simulink model "model_5LinkWalking"  (R2022b)
settings: Solver=ode45  StartTime=0.0  StopTime=Tf  FixedStep=1e-5  MaxStep=1e-3  RelTol=1e-12  AbsTol=1e-8
values from neighbouring files (symbols this model uses):
  f_dist = [0; -100; 0]    [main.m]    (also in main_5linkWalking_PSO.m)
  gains = [ ... (first row only)    [main.m]    (also in main_5linkWalking_PSO.m = [gain.kP1, gain.kD1, gain.kP2, gain.kD2, gain.kP3, gain.kD3,)
  gains_VSLIPSL = [gain_VSLIPSL.K_p; gain_VSLIPSL.K_d; gain_VSLIPSL.K_p_sw; gain_VSLIPSL.K_d_sw; gain_VSLIPSL.K_p_ds; gain_VSLIPSL.K_d_ds; gain_VSLIPSL.K_v_ds]    [main.m]    (also in main_5linkWalking_PSO.m)
  init_flag = [1; 0; -dc.col_param.footPlus; -slipsl.time_ss(N); slipsl.x_ss(1); slipsl.y_ss(1); alpha_ss_ref(1)]    [main.m]    (also in main_5linkWalking_PSO.m = [1; 0; -dc.col_param.footPlus; 0; CoM(1); CoM(2)])
  Initial_state = [q0;dq0]    [main.m]    (also in main_5linkWalking_PSO.m)
  param = [params.m1; params.m2; params.m5; params.l1; params.l2; params.l5; params.g; params.I1; params.I2; params.I5; params.r_k; params.r_h; params.k_ba; params.phi_h0; params.phi_k0]    [main.m]    (also in main_5linkWalking_PSO.m = [params.m1; params.m2; params.m5; params.l1; params.l2; para)
  ref_star_ds = [ref_star.ds.x_CoM_star,      ref_star.ds.y_CoM_star, ref_star.ds.dx_CoM_star,      ref_star.ds.del_y_CoM_star, ref_star.ds.del_dx_CoM_star,      ref_star.ds.del2_y_CoM_star]    [main.m]    (also in main_5linkWalking_PSO.m)
  ref_star_ss = [ref_star.ss.x_M_star,      ref_star.ss.y_M_star, ref_star.ss.x_swFoot_star, ref_star.ss.y_swFoot_star,      ref_star.ss.del_y_M_star, ref_star.ss.del_x_swFoot_star, ref_star.ss.del_y_swFoot_star,      ref_star.ss.del2_y_M_star, ref_star.ss.del2_x_swFoot_star, ref_star.ss.del2_y_swFoot_star,      ref_star.ss.x_CoM_star]    [main.m]    (also in main_5linkWalking_PSO.m)
  sample_time = 0.001    [main.m]    (also in main_5linkWalking_PSO.m)
  slipslParams = [ ... (first row only)    [main.m]    (also in main_5linkWalking_PSO.m)
  slipslTraj_ds = [slipsl.time_ds, slipsl.x_ds, slipsl.y_ds, slipsl.dx_ds, slipsl.dy_ds, alpha_ds_ref_discrete]    [main.m]    (also in main_5linkWalking_PSO.m = [ref_star.dc.ds.time - ref_star.dc.ds.time(1), ref_star.dc.d)
  slipslTraj_ss = [slipsl.time_ss, slipsl.x_ss, slipsl.y_ss, slipsl.dx_ss, slipsl.dy_ss, alpha_ss_ref_discrete]    [main.m]    (also in main_5linkWalking_PSO.m = [ref_star.dc.ss.time, ref_star.dc.ss.x_CoM', ref_star.dc.ss.)
  swFootTraj = [swFootSLIPSL.x_CoM, swFootSLIPSL.x, swFootSLIPSL.z, swFootSLIPSL.dx, swFootSLIPSL.dz]    [main.m]    (also in main_5linkWalking_PSO.m = [ref_star.dc.ss.x_CoM', ref_star.dc.ss.x_sw', ref_star.dc.ss)
libraries: simulink x1
(part 3 of 3)

== matlab function model_5LinkWalking/Model dynamics/STOP system when dx_CoM<=0/MATLAB Function ==
  data: u input
function fcn(u)
if u ~= 0
    disp('dx < 0')
end

== matlab function model_5LinkWalking/Model dynamics/Continuous dynamics ==
  data: t input; U input; dX output; rec_cs_force output; X input; param input; flg_VLO output; flag input; CoM_acc output; f_dist input
function [dX, rec_cs_force, flg_VLO, CoM_acc] = fcn(t, U, X, param, flag, f_dist)

%% variables
th1 = X(1);
th2 = X(2);
th3 = X(3);
th4 = X(4);
th5 = X(5);

dth1 = X(6);
dth2 = X(7);
dth3 = X(8);
dth4 = X(9);
dth5 = X(10);

q = [th1;th2;th3;th4;th5];
dq = [dth1;dth2;dth3;dth4;dth5];

%% parameters

m1 = param(1);
m2 = param(2);
m3 = m2;
m4 = m1;
m5 = param(3);

l1 = param(4);
l2 = param(5);
l5 = param(6);
l3 = l2;
l4 = l1;

gravi = param(7);
I1 = param(8);
I2 = param(9);
I5 = param(10);
I3 = I1;
I4 = I2;

%% flags
f_SS = flag(1); % indicates which stance phase it is
foot = flag(2); % location of the stance foot
foot_prev = flag(3); % previous location of the stance foot

%% Inertia Matrix
MM = MM_matrix(X,param);

%% Centrifugal force · Coriolis force Vector
CC = zeros(5,1);

CC(1, 1) = - (dth2^2*l1*l3*m3*sin(th2 + th3))/2 - dth2^2*l1*l3*m4*sin(th2 + th3) - (dth3^2*l1*l3*m3*sin(th2 + th3))/2 - dth3^2*l1*l3*m4*sin(th2 + th3) - (dth2^2*l1*l5*m5*sin(th2 + th5))/2 - (dth3^2*l2*l4*m4*sin(th3 + th4))/2 - (dth4^2*l2*l4*m4*sin(th3 + th4))/2 - (dth5^2*l1*l5*m5*sin(th2 + th5))/2 - (dth2^2*l1*l2*m2*sin(th2))/2 - dth2^2*l1*l2*m3*sin(th2) - dth2^2*l1*l2*m4*sin(th2) - dth2^2*l1*l2*m5*sin(th2) - (dth3^2*l2*l3*m3*sin(th3))/2 - dth3^2*l2*l3*m4*sin(th3) - (dth4^2*l3*l4*m4*sin(th4))/2 - (dth5^2*l2*l5*m5*sin(th5))/2 - (dth2^2*l1*l4*m4*sin(th2 + th3 + th4))/2 - (dth3^2*l1*l4*m4*sin(th2 + th3 + th4))/2 - (dth4^2*l1*l4*m4*sin(th2 + th3 + th4))/2 - dth1*dth2*l1*l3*m3*sin(th2 + th3) - 2*dth1*dth2*l1*l3*m4*sin(th2 + th3) - dth1*dth3*l1*l3*m3*sin(th2 + th3) - 2*dth1*dth3*l1*l3*m4*sin(th2 + th3) - dth2*dth3*l1*l3*m3*sin(th2 + th3) - 2*dth2*dth3*l1*l3*m4*sin(th2 + th3) - dth1*dth2*l1*l5*m5*sin(th2 + th5) - dth1*dth3*l2*l4*m4*sin(th3 + th4) - dth1*dth4*l2*l4*m4*sin(th3 + th4) - dth2*dth3*l2*l4*m4*sin(th3 + th4) - dth2*dth4*l2*l4*m4*sin(th3 + th4) - dth1*dth5*l1*l5*m5*sin(th2 + th5) - dth3*dth4*l2*l4*m4*sin(th3 + th4) - dth2*dth5*l1*l5*m5*sin(th2 + th5) - dth1*dth2*l1*l2*m2*sin(th2) - 2*dth1*dth2*l1*l2*m3*sin(th2) - 2*dth1*dth2*l1*l2*m4*sin(th2) - 2*dth1*dth2*l1*l2*m5*sin(th2) - dth1*dth3*l2*l3*m3*sin(th3) - 2*dth1*dth3*l2*l3*m4*sin(th3) - dth2*dth3*l2*l3*m3*sin(th3) - 2*dth2*dth3*l2*l3*m4*sin(th3) - dth1*dth4*l3*l4*m4*sin(th4) - dth2*dth4*l3*l4*m4*sin(th4) - dth3*dth4*l3*l4*m4*sin(th4) - dth1*dth5*l2*l5*m5*sin(th5) - dth2*dth5*l2*l5*m5*sin(th5) - dth1*dth2*l1*l4*m4*sin(th2 + th3 + th4) - dth1*dth3*l1*l4*m4*sin(th2 + th3 + th4) - dth1*dth4*l1*l4*m4*sin(th2 + th3 + th4) - dth2*dth3*l1*l4*m4*sin(th2 + th3 + th4) - dth2*dth4*l1*l4*m4*sin(th2 + th3 + th4) - dth3*dth4*l1*l4*m4*sin(th2 + th3 + th4);
CC(2, 1) = (dth1^2*l1*l3*m3*sin(th2 + th3))/2 + dth1^2*l1*l3*m4*sin(th2 + th3) + (dth1^2*l1*l5*m5*sin(th2 + th5))/2 - (dth3^2*l2*l4*m4*sin(th3 + th4))/2 - (dth4^2*l2*l4*m4*sin(th3 + th4))/2 + (dth1^2*l1*l2*m2*sin(th2))/2 + dth1^2*l1*l2*m3*sin(th2) + dth1^2*l1*l2*m4*sin(th2) + dth1^2*l1*l2*m5*sin(th2) - (dth3^2*l2*l3*m3*sin(th3))/2 - dth3^2*l2*l3*m4*sin(th3) - (dth4^2*l3*l4*m4*sin(th4))/2 - (dth5^2*l2*l5*m5*sin(th5))/2 + (dth1^2*l1*l4*m4*sin(th2 + th3 + th4))/2 - dth1*dth3*l2*l4*m4*sin(th3 + th4) - dth1*dth4*l2*l4*m4*sin(th3 + th4) - dth2*dth3*l2*l4*m4*sin(th3 + th4) - dth2*dth4*l2*l4*m4*sin(th3 + th4) - dth3*dth4*l2*l4*m4*sin(th3 + th4) - dth1*dth3*l2*l3*m3*sin(th3) - 2*dth1*dth3*l2*l3*m4*sin(th3) - dth2*dth3*l2*l3*m3*sin(th3) - 2*dth2*dth3*l2*l3*m4*sin(th3) - dth1*dth4*l3*l4*m4*sin(th4) - dth2*dth4*l3*l4*m4*sin(th4) - dth3*dth4*l3*l4*m4*sin(th4) - dth1*dth5*l2*l5*m5*sin(th5) - dth2*dth5*l2*l5*m5*sin(th5);
CC(3, 1) = (dth1^2*l1*l3*m3*sin(th2 + th3))/2 + dth1^2*l1*l3*m4*sin(th2 + th3) + (dth1^2*l2*l4*m4*sin(th3 + th4))/2 + (dth2^2*l2*l4*m4*sin(th3 + th4))/2 + (dth1^2*l2*l3*m3*sin(th3))/2 + dth1^2*l2*l3*m4*sin(th3) + (dth2^2*l2*l3*m3*sin(th3))/2 + dth2^2*l2*l3*m4*sin(th3) - (dth4^2*l3*l4*m4*sin(th4))/2 + (dth1^2*l1*l4*m4*sin(th2 + th3 + th4))/2 + dth1*dth2*l2*l4*m4*sin(th3 + th4) + dth1*dth2*l2*l3*m3*sin(th3) + 2*dth1*dth2*l2*l3*m4*sin(th3) - dth1*dth4*l3*l4*m4*sin(th4) - dth2*dth4*l3*l4*m4*sin(th4) - dth3*dth4*l3*l4*m4*sin(th4);
CC(4, 1) = (l4*m4*(dth1^2*l2*sin(th3 + th4) + dth2^2*l2*sin(th3 + th4) + dth1^2*l3*sin(th4) + dth2^2*l3*sin(th4) + dth3^2*l3*sin(th4) + dth1^2*l1*sin(th2 + th3 + th4) + 2*dth1*dth2*l2*sin(th3 + th4) + 2*dth1*dth2*l3*sin(th4) + 2*dth1*dth3*l3*sin(th4) + 2*dth2*dth3*l3*sin(th4)))/2;
CC(5, 1) = (l5*m5*(dth1^2*l1*sin(th2 + th5) + dth1^2*l2*sin(th5) + dth2^2*l2*sin(th5) + 2*dth1*dth2*l2*sin(th5)))/2;

%% Gravity Vector
GG = zeros(5,1);

GG(1, 1) = (m3*(l2*cos(th1 + th2) + l1*cos(th1) + (l3*cos(th1 + th2 + th3))/2) + m5*(l2*cos(th1 + th2) + l1*cos(th1) + (l5*cos(th1 + th2 + th5))/2) + m2*((l2*cos(th1 + th2))/2 + l1*cos(th1)) + m4*((l4*cos(th1 + th2 + th3 + th4))/2 + l2*cos(th1 + th2) + l1*cos(th1) + l3*cos(th1 + th2 + th3)) + (l1*m1*cos(th1))/2)*gravi;
GG(2, 1) = (m3*(l2*cos(th1 + th2) + (l3*cos(th1 + th2 + th3))/2) + m5*(l2*cos(th1 + th2) + (l5*cos(th1 + th2 + th5))/2) + m4*((l4*cos(th1 + th2 + th3 + th4))/2 + l2*cos(th1 + th2) + l3*cos(th1 + th2 + th3)) + (l2*m2*cos(th1 + th2))/2)*gravi;
GG(3, 1) = (m4*((l4*cos(th1 + th2 + th3 + th4))/2 + l3*cos(th1 + th2 + th3)) + (l3*m3*cos(th1 + th2 + th3))/2)*gravi;
GG(4, 1) = ((l4*m4*cos(th1 + th2 + th3 + th4))/2)*gravi;
GG(5, 1) = ((l5*m5*cos(th1 + th2 + th5))/2)*gravi;

%% input torques mapping matrix
S = [
    1,0,0,0,0;
    0,1,0,0,0;
    0,0,1,0,0;
    0,0,0,1,0;
    0,0,-1,0,1;];

%% Constraint Force Calculation (in case of Double Stance)
J_c = zeros(2,5);
J_c(1,1) = - l4*sin(th1 + th2 + th3 + th4) - l3*sin(th1 + th2 + th3) - l2*sin(th1 + th2) - l1*sin(th1);
J_c(1,2) = - l4*sin(th1 + th2 + th3 + th4) - l3*sin(th1 + th2 + th3) - l2*sin(th1 + th2);
J_c(1,3) = - l4*sin(th1 + th2 + th3 + th4) - l3*sin(th1 + th2 + th3);
J_c(1,4) = - l4*sin(th1 + th2 + th3 + th4);
J_c(1,5) = 0;

J_c(2,1) = l4*cos(th1 + th2 + th3 + th4) + l2*cos(th1 + th2) + l1*cos(th1) + l3*cos(th1 + th2 + th3);
J_c(2,2) = l4*cos(th1 + th2 + th3 + th4) + l2*cos(th1 + th2) + l3*cos(th1 + th2 + th3);
J_c(2,3) = l4*cos(th1 + th2 + th3 + th4) + l3*cos(th1 + th2 + th3);
J_c(2,4) = l4*cos(th1 + th2 + th3 + th4);
J_c(2,5) = 0;

dJ_c = zeros(2,5);
dJ_c(1,1) = - dth3*(l4*cos(th1 + th2 + th3 + th4) + l3*cos(th1 + th2 + th3)) - dth1*(l4*cos(th1 + th2 + th3 + th4) + l2*cos(th1 + th2) + l1*cos(th1) + l3*cos(th1 + th2 + th3)) - dth2*(l4*cos(th1 + th2 + th3 + th4) + l2*cos(th1 + th2) + l3*cos(th1 + th2 + th3)) - dth4*l4*cos(th1 + th2 + th3 + th4);
dJ_c(1,2) = - dth3*(l4*cos(th1 + th2 + th3 + th4) + l3*cos(th1 + th2 + th3)) - dth1*(l4*cos(th1 + th2 + th3 + th4) + l2*cos(th1 + th2) + l3*cos(th1 + th2 + th3)) - dth2*(l4*cos(th1 + th2 + th3 + th4) + l2*cos(th1 + th2) + l3*cos(th1 + th2 + th3)) - dth4*l4*cos(th1 + th2 + th3 + th4);
dJ_c(1,3) = - dth1*(l4*cos(th1 + th2 + th3 + th4) + l3*cos(th1 + th2 + th3)) - dth2*(l4*cos(th1 + th2 + th3 + th4) + l3*cos(th1 + th2 + th3)) - dth3*(l4*cos(th1 + th2 + th3 + th4) + l3*cos(th1 + th2 + th3)) - dth4*l4*cos(th1 + th2 + th3 + th4);
dJ_c(1,4) = - l4*cos(th1 + th2 + th3 + th4)*(dth1 + dth2 + dth3 + dth4);
dJ_c(1,5) = 0;

dJ_c(2,1) = - dth2*(l4*sin(th1 + th2 + th3 + th4) + l2*sin(th1 + th2) + l3*sin(th1 + th2 + th3)) - dth3*(l4*sin(th1 + th2 + th3 + th4) + l3*sin(th1 + th2 + th3)) - dth1*(l4*sin(th1 + th2 + th3 + th4) + l2*sin(th1 + th2) + l1*sin(th1) + l3*sin(th1 + th2 + th3)) - dth4*l4*sin(th1 + th2 + th3 + th4);
dJ_c(2,2) = - dth1*(l4*sin(th1 + th2 + th3 + th4) + l2*sin(th1 + th2) + l3*sin(th1 + th2 + th3)) - dth2*(l4*sin(th1 + th2 + th3 + th4) + l2*sin(th1 + th2) + l3*sin(th1 + th2 + th3)) - dth3*(l4*sin(th1 + th2 + th3 + th4) + l3*sin(th1 + th2 + th3)) - dth4*l4*sin(th1 + th2 + th3 + th4);
dJ_c(2,3) = - dth1*(l4*sin(th1 + th2 + th3 + th4) + l3*sin(th1 + th2 + th3)) - dth2*(l4*sin(th1 + th2 + th3 + th4) + l3*sin(th1 + th2 + th3)) - dth3*(l4*sin(th1 + th2 + th3 + th4) + l3*sin(th1 + th2 + th3)) - dth4*l4*sin(th1 + th2 + th3 + th4);
dJ_c(2,4) = - l4*sin(th1 + th2 + th3 + th4)*(dth1 + dth2 + dth3 + dth4);
dJ_c(2,5) = 0;

constraint_force = zeros(2,1);
constraint_force = -inv(J_c*inv(MM)*J_c')*(J_c*inv(MM)*(S*U-CC-GG)+dJ_c*dq);

%% Disturbance

flag_dist = f_dist(1);
F_dist_x = f_dist(2);
F_dist_y = f_dist(3);

J_dist = [
    - l2*sin(th1 + th2) - l1*sin(th1), -l2*sin(th1 + th2), 0, 0, 0;
      l2*cos(th1 + th2) + l1*cos(th1),  l2*cos(th1 + th2), 0, 0, 0];

%% Acceleration Calculation
ddq = zeros(5,1);
rec_cs_force = [0;0;0;0];

switch_time = flag(4); % time when double stance phase begins

if flag_dist == 1 && (t >= 10 && t <=10.1)
    % if the disturbance is enabled
    if (f_SS == -1 && constraint_force(2) >= 0) || (f_SS == -1 && t - switch_time < 0.05) % second part is because right after impact, there might be some fluctuations so it disregards them for 0.01 secs
        % if f_SS == 0
        ddq = inv(MM)*(- CC - GG + S*U + transpose(J_c)*constraint_force + transpose(J_dist)*[F_dist_x; F_dist_y]);
        rec_cs_force = [constraint_force; 0;0];
    else
        rec_cs_force = [0; 0; constraint_force];
        constraint_force = [0; 0]; % don't constraint the swing foot if force in horizontal direction is pulling if its not right after the impact
        ddq = inv(MM)*(- CC - GG + S*U + transpose(J_dist)*[F_dist_x; F_dist_y]);
    end
else
    % if the disturbance is disabled
    if (f_SS == -1 && constraint_force(2) >= 0) || (f_SS == -1 && t - switch_time < 0.05) % second part is because right after impact, there might be some fluctuations so it disregards them for 0.01 secs
        % if f_SS == 0
        ddq = inv(MM)*(- CC - GG + S*U + transpose(J_c)*constraint_force);
        rec_cs_force = [constraint_force; 0;0];
    else
        rec_cs_force = [0; 0; constraint_force];
        constraint_force = [0; 0]; % don't constraint the swing foot if force in horizontal direction is pulling if its not right after the impact
        ddq = inv(MM)*(- CC - GG + S*U);
    end
end


%% VLO Detection

CoM = calculate_com(X, param, 0, [0;0;0;0;0]); % calculation the CoM location
if CoM(1) >= 0
    flg_VLO = 1;
else
    flg_VLO = 0;
end

%% Acceleration of CoM to visualize tracking of desired CoM acc.
ddth1 = ddq(1);
ddth2 = ddq(2);
ddth3 = ddq(3);
ddth4 = ddq(4);
ddth5 = ddq(5);

x1 = foot;
xG = (m4*(x1 + (l4*cos(th1 + th2 + th3 + th4))/2 + l2*cos(th1 + th2) + l1*cos(th1) + l3*cos(th1 + th2 + th3)) + m1*(x1 + (l1*cos(th1))/2) + m3*(x1 + l2*cos(th1 + th2) + l1*cos(th1) + (l3*cos(th1 + th2 + th3))/2) + m5*(x1 + l2*cos(th1 + th2) + l1*cos(th1) + (l5*cos(th1 + th2 + th5))/2) + m2*(x1 + (l1*cos(th1 + th2))/2 + l1*cos(th1)))/(m1 + m2 + m3 + m4 + m5);
zG = (m3*(l2*sin(th1 + th2) + l1*sin(th1) + (l3*sin(th1 + th2 + th3))/2) + m5*(l2*sin(th1 + th2) + l1*sin(th1) + (l5*sin(th1 + th2 + th5))/2) + m2*((l2*sin(th1 + th2))/2 + l1*sin(th1)) + m4*((l4*sin(th1 + th2 + th3 + th4))/2 + l2*sin(th1 + th2) + l1*sin(th1) + l3*sin(th1 + th2 + th3)) + (l1*m1*sin(th1))/2)/(m1 + m2 + m3 + m4 + m5);

dxG = - (dth3*(m4*((l4*sin(th1 + th2 + th3 + th4))/2 + l3*sin(th1 + th2 + th3)) + (l3*m3*sin(th1 + th2 + th3))/2))/(m1 + m2 + m3 + m4 + m5) - (dth1*(m3*(l2*sin(th1 + th2) + l1*sin(th1) + (l3*sin(th1 + th2 + th3))/2) + m5*(l2*sin(th1 + th2) + l1*sin(th1) + (l5*sin(th1 + th2 + th5))/2) + m2*((l1*sin(th1 + th2))/2 + l1*sin(th1)) + m4*((l4*sin(th1 + th2 + th3 + th4))/2 + l2*sin(th1 + th2) + l1*sin(th1) + l3*sin(th1 + th2 + th3)) + (l1*m1*sin(th1))/2))/(m1 + m2 + m3 + m4 + m5) - (dth2*(m4*((l4*sin(th1 + th2 + th3 + th4))/2 + l2*sin(th1 + th2) + l3*sin(th1 + th2 + th3)) + m3*(l2*sin(th1 + th2) + (l3*sin(th1 + th2 + th3))/2) + m5*(l2*sin(th1 + th2) + (l5*sin(th1 + th2 + th5))/2) + (l1*m2*sin(th1 + th2))/2))/(m1 + m2 + m3 + m4 + m5) - (dth4*l4*m4*sin(th1 + th2 + th3 + th4))/(2*(m1 + m2 + m3 + m4 + m5)) - (dth5*l5*m5*sin(th1 + th2 + th5))/(2*(m1 + m2 + m3 + m4 + m5));
dzG = (dth1*(m3*(l2*cos(th1 + th2) + l1*cos(th1) + (l3*cos(th1 + th2 + th3))/2) + m5*(l2*cos(th1 + th2) + l1*cos(th1) + (l5*cos(th1 + th2 + th5))/2) + m2*((l2*cos(th1 + th2))/2 + l1*cos(th1)) + m4*((l4*cos(th1 + th2 + th3 + th4))/2 + l2*cos(th1 + th2) + l1*cos(th1) + l3*cos(th1 + th2 + th3)) + (l1*m1*cos(th1))/2))/(m1 + m2 + m3 + m4 + m5) + (dth3*(m4*((l4*cos(th1 + th2 + th3 + th4))/2 + l3*cos(th1 + th2 + th3)) + (l3*m3*cos(th1 + th2 + th3))/2))/(m1 + m2 + m3 + m4 + m5) + (dth2*(m3*(l2*cos(th1 + th2) + (l3*cos(th1 + th2 + th3))/2) + m5*(l2*cos(th1 + th2) + (l5*cos(th1 + th2 + th5))/2) + m4*((l4*cos(th1 + th2 + th3 + th4))/2 + l2*cos(th1 + th2) + l3*cos(th1 + th2 + th3)) + (l2*m2*cos(th1 + th2))/2))/(m1 + m2 + m3 + m4 + m5) + (dth4*l4*m4*cos(th1 + th2 + th3 + th4))/(2*(m1 + m2 + m3 + m4 + m5)) + (dth5*l5*m5*cos(th1 + th2 + th5))/(2*(m1 + m2 + m3 + m4 + m5));

ddxG = - dth4*((dth1*l4*m4*cos(th1 + th2 + th3 + th4))/(2*(m1 + m2 + m3 + m4 + m5)) + (dth2*l4*m4*cos(th1 + th2 + th3 + th4))/(2*(m1 + m2 + m3 + m4 + m5)) + (dth3*l4*m4*cos(th1 + th2 + th3 + th4))/(2*(m1 + m2 + m3 + m4 + m5)) + (dth4*l4*m4*cos(th1 + th2 + th3 + th4))/(2*(m1 + m2 + m3 + m4 + m5))) - dth2*((dth3*(m4*((l4*cos(th1 + th2 + th3 + th4))/2 + l3*cos(th1 + th2 + th3)) + (l3*m3*cos(th1 + th2 + th3))/2))/(m1 + m2 + m3 + m4 + m5) + (dth1*(m3*(l2*cos(th1 + th2) + (l3*cos(th1 + th2 + th3))/2) + m5*(l2*cos(th1 + th2) + (l5*cos(th1 + th2 + th5))/2) + m4*((l4*cos(th1 + th2 + th3 + th4))/2 + l2*cos(th1 + th2) + l3*cos(th1 + th2 + th3)) + (l1*m2*cos(th1 + th2))/2))/(m1 + m2 + m3 + m4 + m5) + (dth2*(m3*(l2*cos(th1 + th2) + (l3*cos(th1 + th2 + th3))/2) + m5*(l2*cos(th1 + th2) + (l5*cos(th1 + th2 + th5))/2) + m4*((l4*cos(th1 + th2 + th3 + th4))/2 + l2*cos(th1 + th2) + l3*cos(th1 + th2 + th3)) + (l1*m2*cos(th1 + th2))/2))/(m1 + m2 + m3 + m4 + m5) + (dth4*l4*m4*cos(th1 + th2 + th3 + th4))/(2*(m1 + m2 + m3 + m4 + m5)) + (dth5*l5*m5*cos(th1 + th2 + th5))/(2*(m1 + m2 + m3 + m4 + m5))) - dth3*((dth1*(m4*((l4*cos(th1 + th2 + th3 + th4))/2 + l3*cos(th1 + th2 + th3)) + (l3*m3*cos(th1 + th2 + th3))/2))/(m1 + m2 + m3 + m4 + m5) + (dth2*(m4*((l4*cos(th1 + th2 + th3 + th4))/2 + l3*cos(th1 + th2 + th3)) + (l3*m3*cos(th1 + th2 + th3))/2))/(m1 + m2 + m3 + m4 + m5) + (dth3*(m4*((l4*cos(th1 + th2 + th3 + th4))/2 + l3*cos(th1 + th2 + th3)) + (l3*m3*cos(th1 + th2 + th3))/2))/(m1 + m2 + m3 + m4 + m5) + (dth4*l4*m4*cos(th1 + th2 + th3 + th4))/(2*(m1 + m2 + m3 + m4 + m5))) - dth1*((dth1*(m3*(l2*cos(th1 + th2) + l1*cos(th1) + (l3*cos(th1 + th2 + th3))/2) + m5*(l2*cos(th1 + th2) + l1*cos(th1) + (l5*cos(th1 + th2 + th5))/2) + m2*((l1*cos(th1 + th2))/2 + l1*cos(th1)) + m4*((l4*cos(th1 + th2 + th3 + th4))/2 + l2*cos(th1 + th2) + l1*cos(th1) + l3*cos(th1 + th2 + th3)) + (l1*m1*cos(th1))/2))/(m1 + m2 + m3 + m4 + m5) + (dth3*(m4*((l4*cos(th1 + th2 + th3 + th4))/2 + l3*cos(th1 + th2 + th3)) + (l3*m3*cos(th1 + th2 + th3))/2))/(m1 + m2 + m3 + m4 + m5) + (dth2*(m3*(l2*cos(th1 + th2) + (l3*cos(th1 + th2 + th3))/2) + m5*(l2*cos(th1 + th2) + (l5*cos(th1 + th2 + th5))/2) + m4*((l4*cos(th1 + th2 + th3 + th4))/2 + l2*cos(th1 + th2) + l3*cos(th1 + th2 + th3)) + (l1*m2*cos(th1 + th2))/2))/(m1 + m2 + m3 + m4 + m5) + (dth4*l4*m4*cos(th1 + th2 + th3 + th4))/(2*(m1 + m2 + m3 + m4 + m5)) + (dth5*l5*m5*cos(th1 + th2 + th5))/(2*(m1 + m2 + m3 + m4 + m5))) - dth5*((dth1*l5*m5*cos(th1 + th2 + th5))/(2*(m1 + m2 + m3 + m4 + m5)) + (dth2*l5*m5*cos(th1 + th2 + th5))/(2*(m1 + m2 + m3 + m4 + m5)) + (dth5*l5*m5*cos(th1 + th2 + th5))/(2*(m1 + m2 + m3 + m4 + m5))) - (ddth3*(m4*((l4*sin(th1 + th2 + th3 + th4))/2 + l3*sin(th1 + th2 + th3)) + (l3*m3*sin(th1 + th2 + th3))/2))/(m1 + m2 + m3 + m4 + m5) - (ddth1*(m3*(l2*sin(th1 + th2) + l1*sin(th1) + (l3*sin(th1 + th2 + th3))/2) + m5*(l2*sin(th1 + th2) + l1*sin(th1) + (l5*sin(th1 + th2 + th5))/2) + m2*((l1*sin(th1 + th2))/2 + l1*sin(th1)) + m4*((l4*sin(th1 + th2 + th3 + th4))/2 + l2*sin(th1 + th2) + l1*sin(th1) + l3*sin(th1 + th2 + th3)) + (l1*m1*sin(th1))/2))/(m1 + m2 + m3 + m4 + m5) - (ddth2*(m4*((l4*sin(th1 + th2 + th3 + th4))/2 + l2*sin(th1 + th2) + l3*sin(th1 + th2 + th3)) + m3*(l2*sin(th1 + th2) + (l3*sin(th1 + th2 + th3))/2) + m5*(l2*sin(th1 + th2) + (l5*sin(th1 + th2 + th5))/2) + (l1*m2*sin(th1 + th2))/2))/(m1 + m2 + m3 + m4 + m5) - (ddth4*l4*m4*sin(th1 + th2 + th3 + th4))/(2*(m1 + m2 + m3 + m4 + m5)) - (ddth5*l5*m5*sin(th1 + th2 + th5))/(2*(m1 + m2 + m3 + m4 + m5));
ddzG = (ddth1*(m3*(l2*cos(th1 + th2) + l1*cos(th1) + (l3*cos(th1 + th2 + th3))/2) + m5*(l2*cos(th1 + th2) + l1*cos(th1) + (l5*cos(th1 + th2 + th5))/2) + m2*((l2*cos(th1 + th2))/2 + l1*cos(th1)) + m4*((l4*cos(th1 + th2 + th3 + th4))/2 + l2*cos(th1 + th2) + l1*cos(th1) + l3*cos(th1 + th2 + th3)) + (l1*m1*cos(th1))/2))/(m1 + m2 + m3 + m4 + m5) - dth3*((dth1*(m4*((l4*sin(th1 + th2 + th3 + th4))/2 + l3*sin(th1 + th2 + th3)) + (l3*m3*sin(th1 + th2 + th3))/2))/(m1 + m2 + m3 + m4 + m5) + (dth2*(m4*((l4*sin(th1 + th2 + th3 + th4))/2 + l3*sin(th1 + th2 + th3)) + (l3*m3*sin(th1 + th2 + th3))/2))/(m1 + m2 + m3 + m4 + m5) + (dth3*(m4*((l4*sin(th1 + th2 + th3 + th4))/2 + l3*sin(th1 + th2 + th3)) + (l3*m3*sin(th1 + th2 + th3))/2))/(m1 + m2 + m3 + m4 + m5) + (dth4*l4*m4*sin(th1 + th2 + th3 + th4))/(2*(m1 + m2 + m3 + m4 + m5))) - dth1*((dth3*(m4*((l4*sin(th1 + th2 + th3 + th4))/2 + l3*sin(th1 + th2 + th3)) + (l3*m3*sin(th1 + th2 + th3))/2))/(m1 + m2 + m3 + m4 + m5) + (dth1*(m3*(l2*sin(th1 + th2) + l1*sin(th1) + (l3*sin(th1 + th2 + th3))/2) + m5*(l2*sin(th1 + th2) + l1*sin(th1) + (l5*sin(th1 + th2 + th5))/2) + m2*((l2*sin(th1 + th2))/2 + l1*sin(th1)) + m4*((l4*sin(th1 + th2 + th3 + th4))/2 + l2*sin(th1 + th2) + l1*sin(th1) + l3*sin(th1 + th2 + th3)) + (l1*m1*sin(th1))/2))/(m1 + m2 + m3 + m4 + m5) + (dth2*(m4*((l4*sin(th1 + th2 + th3 + th4))/2 + l2*sin(th1 + th2) + l3*sin(th1 + th2 + th3)) + m3*(l2*sin(th1 + th2) + (l3*sin(th1 + th2 + th3))/2) + m5*(l2*sin(th1 + th2) + (l5*sin(th1 + th2 + th5))/2) + (l2*m2*sin(th1 + th2))/2))/(m1 + m2 + m3 + m4 + m5) + (dth4*l4*m4*sin(th1 + th2 + th3 + th4))/(2*(m1 + m2 + m3 + m4 + m5)) + (dth5*l5*m5*sin(th1 + th2 + th5))/(2*(m1 + m2 + m3 + m4 + m5))) - dth4*((dth1*l4*m4*sin(th1 + th2 + th3 + th4))/(2*(m1 + m2 + m3 + m4 + m5)) + (dth2*l4*m4*sin(th1 + th2 + th3 + th4))/(2*(m1 + m2 + m3 + m4 + m5)) + (dth3*l4*m4*sin(th1 + th2 + th3 + th4))/(2*(m1 + m2 + m3 + m4 + m5)) + (dth4*l4*m4*sin(th1 + th2 + th3 + th4))/(2*(m1 + m2 + m3 + m4 + m5))) - dth2*((dth3*(m4*((l4*sin(th1 + th2 + th3 + th4))/2 + l3*sin(th1 + th2 + th3)) + (l3*m3*sin(th1 + th2 + th3))/2))/(m1 + m2 + m3 + m4 + m5) + (dth1*(m4*((l4*sin(th1 + th2 + th3 + th4))/2 + l2*sin(th1 + th2) + l3*sin(th1 + th2 + th3)) + m3*(l2*sin(th1 + th2) + (l3*sin(th1 + th2 + th3))/2) + m5*(l2*sin(th1 + th2) + (l5*sin(th1 + th2 + th5))/2) + (l2*m2*sin(th1 + th2))/2))/(m1 + m2 + m3 + m4 + m5) + (dth2*(m4*((l4*sin(th1 + th2 + th3 + th4))/2 + l2*sin(th1 + th2) + l3*sin(th1 + th2 + th3)) + m3*(l2*sin(th1 + th2) + (l3*sin(th1 + th2 + th3))/2) + m5*(l2*sin(th1 + th2) + (l5*sin(th1 + th2 + th5))/2) + (l2*m2*sin(th1 + th2))/2))/(m1 + m2 + m3 + m4 + m5) + (dth4*l4*m4*sin(th1 + th2 + th3 + th4))/(2*(m1 + m2 + m3 + m4 + m5)) + (dth5*l5*m5*sin(th1 + th2 + th5))/(2*(m1 + m2 + m3 + m4 + m5))) - dth5*((dth1*l5*m5*sin(th1 + th2 + th5))/(2*(m1 + m2 + m3 + m4 + m5)) + (dth2*l5*m5*sin(th1 + th2 + th5))/(2*(m1 + m2 + m3 + m4 + m5)) + (dth5*l5*m5*sin(th1 + th2 + th5))/(2*(m1 + m2 + m3 + m4 + m5))) + (ddth3*(m4*((l4*cos(th1 + th2 + th3 + th4))/2 + l3*cos(th1 + th2 + th3)) + (l3*m3*cos(th1 + th2 + th3))/2))/(m1 + m2 + m3 + m4 + m5) + (ddth2*(m3*(l2*cos(th1 + th2) + (l3*cos(th1 + th2 + th3))/2) + m5*(l2*cos(th1 + th2) + (l5*cos(th1 + th2 + th5))/2) + m4*((l4*cos(th1 + th2 + th3 + th4))/2 + l2*cos(th1 + th2) + l3*cos(th1 + th2 + th3)) + (l2*m2*cos(th1 + th2))/2))/(m1 + m2 + m3 + m4 + m5) + (ddth4*l4*m4*cos(th1 + th2 + th3 + th4))/(2*(m1 + m2 + m3 + m4 + m5)) + (ddth5*l5*m5*cos(th1 + th2 + th5))/(2*(m1 + m2 + m3 + m4 + m5));

CoM_acc = [xG; zG; dxG; dzG; ddxG; ddzG];

%%
dX = [dq; ddq];

end

== matlab function model_5LinkWalking/Model dynamics/STOP system when dx_CoM<=0/MATLAB Function1 ==
  data: X input; param input; flag input; zG output; dxG output; th2 output; th4 output
function [zG, dxG, th2, th4] = fcn(X,param, flag)

%% variables
th1 = X(1);
th2 = X(2);
th3 = X(3);
th4 = X(4);
th5 = X(5);

dth1 = X(6);
dth2 = X(7);
dth3 = X(8);
dth4 = X(9);
dth5 = X(10);

q = [th1;th2;th3;th4;th5];
dq = [dth1;dth2;dth3;dth4;dth5];

%% parameters

m1 = param(1);
m2 = param(2);
m3 = m2;
m4 = m1;
m5 = param(3);

l1 = param(4);
l2 = param(5);
l5 = param(6);
l3 = l2;
l4 = l1;

gravi = param(7);
I1 = param(8);
I2 = param(9);
I5 = param(10);
I3 = I1;
I4 = I2;

k_s = param(11);
r_k = param(12);
r_b = param(13);

%% flags
f_SS = flag(1); % indicates which stance phase it is
foot = flag(2); % location of the stance foot
foot_prev = flag(3); % previous location of the stance foot

%% CoM calculation
% CoM = [xG, zG, dxG, dzG, ddxG, ddzG];
CoM = calculate_com(X, param, 0, [0;0;0;0;0]); % calculation the CoM location

xG = CoM(1);
zG = CoM(2);
dxG = CoM(3);
dzG = CoM(4);

== matlab function model_5LinkWalking/SLIP-SL Controller/SLIP_Controller ==
  settings: updateMethod=DISCRETE
  data: t input; X input; U output; param input; gains input; flag input; des_traj input; flag_des input; des_th input; des_z_dz_dx output; U_test output; x1_prev input; x1_prev output
function [U, des_z_dz_dx, U_test, x1_prev] = fcn(t, X, param, gains,  flag, des_traj, flag_des, des_th, x1_prev)
coder.extrinsic('quadprog');
coder.extrinsic('sparse')

%% variables (absolute angles)
th1 = X(1);
th2 = X(1) + X(2);
th3 = X(1) + X(2) + X(3);
th4 = X(1) + X(2) + X(3) + X(4);
th5 = X(1) + X(2) + X(5);

dth1 = X(6);
dth2 = X(6) + X(7);
dth3 = X(6) + X(7) + X(8);
dth4 = X(6) + X(7) + X(8) + X(9);
dth5 = X(6) + X(7) + X(10);

q = [th1;th2;th3;th4;th5];
dq = [dth1;dth2;dth3;dth4;dth5];

%% Parameters

m1 = param(1);
m2 = param(2);
m3 = m2;
m4 = m1;
m5 = param(3);

l1 = param(4);
l2 = param(5);
l5 = param(6);
l3 = l2;
l4 = l1;

gravi = param(7);
I1 = param(8);
I2 = param(9);
I5 = param(10);
I3 = I1;
I4 = I2;

%% flags
f_SS = flag(1); % indicates which stance phase it is
foot = flag(2); % location of the stance foot
foot_prev = flag(3); % previous location of the stance foot

t_mode_change = flag(4); % time stamp when the mode change happens (TD or LO)

x_LO = flag(5); % lift off location of CoM when it happened

%% Inertia Matrix
MM = MM_matrix_absolute(X,param);

%% Centrifugal force · Coriolis force Vector
CC = zeros(5,1);

CC(1, 1) = (l1*(dth2^2*l2*m2*sin(th1 - th2) + 2*dth2^2*l2*m3*sin(th1 - th2) + 2*dth2^2*l2*m4*sin(th1 - th2) + 2*dth2^2*l2*m5*sin(th1 - th2) + dth3^2*l3*m3*sin(th1 - th3) + 2*dth3^2*l3*m4*sin(th1 - th3) + dth4^2*l4*m4*sin(th1 - th4) + dth5^2*l5*m5*sin(th1 - th5)))/2;
CC(2, 1) = -(l2*(dth1^2*l1*m2*sin(th1 - th2) + 2*dth1^2*l1*m3*sin(th1 - th2) + 2*dth1^2*l1*m4*sin(th1 - th2) + 2*dth1^2*l1*m5*sin(th1 - th2) - dth3^2*l3*m3*sin(th2 - th3) - 2*dth3^2*l3*m4*sin(th2 - th3) - dth4^2*l4*m4*sin(th2 - th4) - dth5^2*l5*m5*sin(th2 - th5)))/2;
CC(3, 1) = -(l3*(dth1^2*l1*m3*sin(th1 - th3) + 2*dth1^2*l1*m4*sin(th1 - th3) + dth2^2*l2*m3*sin(th2 - th3) + 2*dth2^2*l2*m4*sin(th2 - th3) - dth4^2*l4*m4*sin(th3 - th4)))/2;
CC(4, 1) = -(l4*m4*(l1*sin(th1 - th4)*dth1^2 + l2*sin(th2 - th4)*dth2^2 + l3*sin(th3 - th4)*dth3^2))/2;
CC(5, 1) = -(l5*m5*(l1*sin(th1 - th5)*dth1^2 + l2*sin(th2 - th5)*dth2^2))/2;

%% Gravity Vector
GG = zeros(5,1);

GG(1, 1) = (gravi*l1*cos(th1)*(m1 + 2*m2 + 2*m3 + 2*m4 + 2*m5))/2;
GG(2, 1) = (gravi*l2*cos(th2)*(m2 + 2*m3 + 2*m4 + 2*m5))/2;
GG(3, 1) = (gravi*l3*cos(th3)*(m3 + 2*m4))/2;
GG(4, 1) = ((l4*m4*cos(th4))/2)*gravi;
GG(5, 1) = ((l5*m5*cos(th5))/2)*gravi;

%% input torques mapping matrix
S = [
     1,-1, 0, 0, 0;
     0, 1, 0, 0,-1;
     0, 0, 1,-1, 0;
     0, 0, 0, 1, 0;
     0, 0,-1, 0, 1;];

%% Controller Gains
kP1 = gains(1);
kD1 = gains(2);
kP2 = gains(3);
kD2 = gains(4);
kP3 = gains(5);
kD3 = gains(6);
kP4 = gains(7);
kD4 = gains(8);
kP5 = gains(9);
kD5 = gains(10);

%% desired traj and flag

% des_traj

ddx_des = des_traj(1);
ddz_des = des_traj(2);
ddx_sw_ft_des = des_traj(3);
ddz_sw_ft_des = des_traj(4);

dx_des = des_traj(5);
dz_des = des_traj(6);
dx_sw_ft_des = des_traj(7);
dz_sw_ft_des = des_traj(8);

x_des = des_traj(9);
z_des = des_traj(10);
x_sw_ft_des = des_traj(11);
z_sw_ft_des = des_traj(12);

flag_des = flag_des;

%% Joint angle control
th1_des_abs = des_th(1);
th2_des_abs = des_th(1) + des_th(2);
th3_des_abs = des_th(1) + des_th(2) + des_th(3);
th4_des_abs = des_th(1) + des_th(2) + des_th(3) + des_th(4);
th5_des_abs = des_th(1) + des_th(2) + des_th(5);

dth1_des_abs = des_th(6);
dth2_des_abs = des_th(6) + des_th(7);
dth3_des_abs = des_th(6) + des_th(7) + des_th(8);
dth4_des_abs = des_th(6) + des_th(7) + des_th(8) + des_th(9);
dth5_des_abs = des_th(6) + des_th(7) + des_th(10);

ddth1_des_abs = des_th(11);
ddth2_des_abs = des_th(11) + des_th(12);
ddth3_des_abs = des_th(11) + des_th(12) + des_th(13);
ddth4_des_abs = des_th(11) + des_th(12) + des_th(13) + des_th(14);
ddth5_des_abs = des_th(11) + des_th(12) + des_th(15);

ddx_t = zeros(5,1);

ddx_t(1,1) = ddth1_des_abs + kP1*(th1_des_abs - th1) + kD1*(dth1_des_abs - dth1);
ddx_t(2,1) = ddth2_des_abs + kP2*(th2_des_abs - th2) + kD2*(dth2_des_abs - dth2);
ddx_t(3,1) = ddth3_des_abs + kP3*(th3_des_abs - th3) + kD3*(dth3_des_abs - dth3);
ddx_t(4,1) = ddth4_des_abs + kP4*(th4_des_abs - th4) + kD4*(dth4_des_abs - dth4);
ddx_t(5,1) = ddth5_des_abs + kP5*(th5_des_abs - th5) + kD5*(dth5_des_abs - dth5);

% ddx_t(1,1) = kP1*(th1_des_abs - th1) + kD1*(dth1_des_abs - dth1);
% ddx_t(2,1) = kP2*(th2_des_abs - th2) + kD2*(dth2_des_abs - dth2);
% ddx_t(3,1) = kP3*(th3_des_abs - th3) + kD3*(dth3_des_abs - dth3);
% ddx_t(4,1) = kP4*(th4_des_abs - th4) + kD4*(dth4_des_abs - dth4);
% ddx_t(5,1) = kP5*(th5_des_abs - th5) + kD5*(dth5_des_abs - dth5);

% ddx_t(1,1) = kP_G*(th1_des_abs - th1);
% ddx_t(2,1) = kP_G*(th2_des_abs - th2);
% ddx_t(3,1) = kP_G*(th3_des_abs - th3);
% ddx_t(4,1) = kP_G*(th4_des_abs - th4);
% ddx_t(5,1) = kP_G*(th5_des_abs - th5);

% U = inv(S)*ddx_t;

% trying to cancel out unwanted dynamics
U = inv(S)*(MM*ddx_t + CC + GG);

% trying different controllers for DS and SS with unwanted dynamics canceled
if f_SS == 1
    ddx_t_ss = zeros(5,1);
    ddx_t_ss(1,1) = ddth1_des_abs + kP1*(th1_des_abs - th1) + kD1*(dth1_des_abs - dth1);
    ddx_t_ss(2,1) = ddth2_des_abs + kP2*(th2_des_abs - th2) + kD2*(dth2_des_abs - dth2);
    ddx_t_ss(3,1) = ddth3_des_abs + kP3*(th3_des_abs - th3) + kD3*(dth3_des_abs - dth3);
    ddx_t_ss(4,1) = ddth4_des_abs + kP4*(th4_des_abs - th4) + kD4*(dth4_des_abs - dth4);
    ddx_t_ss(5,1) = ddth5_des_abs + kP5*(th5_des_abs - th5) + kD5*(dth5_des_abs - dth5);
    
%     ddx_t_ss(1,1) = kP1*(th1_des_abs - th1) + kD1*(dth1_des_abs - dth1);
%     ddx_t_ss(2,1) = kP2*(th2_des_abs - th2) + kD2*(dth2_des_abs - dth2);
%     ddx_t_ss(3,1) = kP3*(th3_des_abs - th3) + kD3*(dth3_des_abs - dth3);
%     ddx_t_ss(4,1) = kP4*(th4_des_abs - th4) + kD4*(dth4_des_abs - dth4);
%     ddx_t_ss(5,1) = kP5*(th5_des_abs - th5) + kD5*(dth5_des_abs - dth5);
    
    U = inv(S)*(MM*ddx_t_ss + CC + GG);
else
    ddx_t_ds = zeros(3,1);
    ddx_t_ds(1,1) = ddth3_des_abs + kP3*(th3_des_abs - th3) + kD3*(dth3_des_abs - dth3);
    ddx_t_ds(2,1) = ddth4_des_abs + kP4*(th4_des_abs - th4) + kD4*(dth4_des_abs - dth4);
    ddx_t_ds(3,1) = ddth5_des_abs + kP5*(th5_des_abs - th5) + kD5*(dth5_des_abs - dth5);

%     ddx_t_ds(1,1) = kP3*(th3_des_abs - th3) + kD3*(dth3_des_abs - dth3);
%     ddx_t_ds(2,1) = kP4*(th4_des_abs - th4) + kD4*(dth4_des_abs - dth4);
%     ddx_t_ds(3,1) = kP5*(th5_des_abs - th5) + kD5*(dth5_des_abs - dth5);
    
    % J_hip_sw and J_hip_st, jacobians mapping swing and stance leg velocities to hip velocity
    J_hip_st = [
        -l1*sin(th1), -l2*sin(th2);
        l1*cos(th1),  l2*cos(th2)];
    
    J_hip_sw = [
        l3*sin(th3),  l4*sin(th4);
        -l3*cos(th3), -l4*cos(th4)];
    
    dq_a = [dth3; dth4; dth5];
    Gamma = [inv(J_hip_st)*J_hip_sw, zeros(2,1); eye(3,3)];
    % dGamma_st in derive_Jacobian.m
    dGamma = [
        (l3*(dth3*sin(th1 - 2*th2 + th3) - dth1*sin(th1 - 2*th2 + th3) + dth1*sin(th1 - th3) - 2*dth2*sin(th1 - th3) + dth3*sin(th1 - th3)))/(l1*(cos(2*th1 - 2*th2) - 1)), (l4*(dth4*sin(th1 - 2*th2 + th4) - dth1*sin(th1 - 2*th2 + th4) + dth1*sin(th1 - th4) - 2*dth2*sin(th1 - th4) + dth4*sin(th1 - th4)))/(l1*(cos(2*th1 - 2*th2) - 1)), 0;
        (l3*(dth3*sin(th2 - 2*th1 + th3) - dth2*sin(th2 - 2*th1 + th3) - 2*dth1*sin(th2 - th3) + dth2*sin(th2 - th3) + dth3*sin(th2 - th3)))/(l2*(cos(2*th1 - 2*th2) - 1)), (l4*(dth4*sin(th2 - 2*th1 + th4) - dth2*sin(th2 - 2*th1 + th4) - 2*dth1*sin(th2 - th4) + dth2*sin(th2 - th4) + dth4*sin(th2 - th4)))/(l2*(cos(2*th1 - 2*th2) - 1)), 0;
        zeros(3,3)];
    
    % derivation and definitions are in One Note\Research Diary\5 Link
    % Biarticular Walking\Modifying the 5 Link Simulator
    MM_a = transpose(Gamma)*MM*Gamma;
    CC_a = transpose(Gamma)*MM*dGamma;
    GG_a = transpose(Gamma)*(CC + GG);
    
    % equation (20) from the paper but modified for DS:
    u_a = MM_a*ddx_t_ds + CC_a*dq_a + GG_a;
    
    % weights matrix
    W = eye(5,5);
    W(1,1) = 1;
    W(3,3) = 1;
    W(4,4) = 1;
    
    Gamma_T_W = inv(W)*Gamma*inv(Gamma'*inv(W)*Gamma); % weighted inverse on Gamma transpose
    U = inv(S)*(Gamma_T_W*u_a);
end

%% input saturation
U(1) = sign(U(1))*min(abs(U(1)), 200);
U(2) = sign(U(2))*min(abs(U(2)), 200);
U(3) = sign(U(3))*min(abs(U(3)), 200);
U(4) = sign(U(4))*min(abs(U(4)), 200);
U(5) = sign(U(5))*min(abs(U(5)), 200);

%%
des_z_dz_dx = [x_des; z_des; dx_des; dz_des; ddx_des; ddz_des; flag_des]; % desired acceleration

%% ZMP Control

% U_test = ZMP_control(t, X, param, flag, U);
U_test = [0;0;0;0;0];
% lambda_y = 0;

end
